simulink model "es2_emg_2"  (R2024a)
settings: Solver=VariableStepAuto  StartTime=0.0  StopTime=30  RelTol=1e-3
libraries: vrlib x2
settings Model: Creator=amisq  LastModifiedBy=amisq

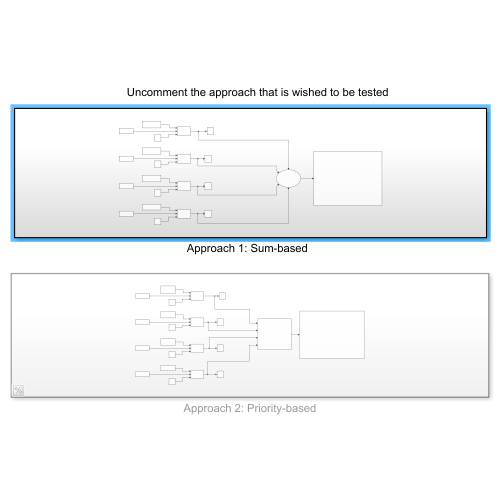
[thumbnail: Simulink's stored preview of the top-level diagram]
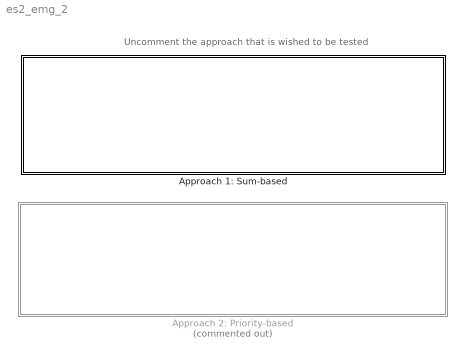
== system es2_emg_2 ==
  note: Uncomment the approach that is wished to be tested
  "Approach 1: Sum-based  " : Subsystem
  Approach 2: Priority-based : Subsystem  Commented=on

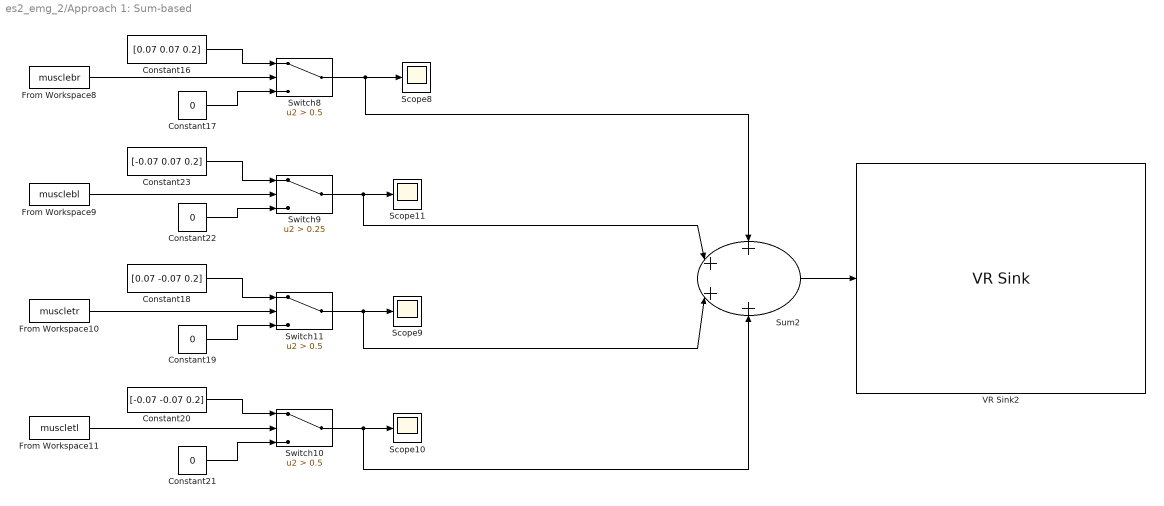
== system es2_emg_2/Approach 1: Sum-based   ==
  Constant16 : Constant  Value=[0.07 0.07 0.2]
  Constant{17,19,21..22} (4 alike) : Constant  Value=0
  Constant18 : Constant  Value=[0.07 -0.07 0.2]
  Constant20 : Constant  Value=[-0.07 -0.07 0.2]
  Constant23 : Constant  Value=[-0.07 0.07 0.2]
  From Workspace10 : FromWorkspace  VariableName=muscletr  SampleTime=0.05
  From Workspace11 : FromWorkspace  VariableName=muscletl  SampleTime=0.05
  From Workspace8 : FromWorkspace  VariableName=musclebr  SampleTime=0.05
  From Workspace9 : FromWorkspace  VariableName=musclebl  SampleTime=0.05
  Scope{8..11} (4 alike) : Scope
  Sum2 : Sum  Inputs=++++
  Switch10 : Switch  Criteria=u2 > Threshold  Threshold=0.5  SaturateOnIntegerOverflow=off  InputSameDT=off
  Switch11 : Switch  Criteria=u2 > Threshold  Threshold=0.5  SaturateOnIntegerOverflow=off  InputSameDT=off
  Switch8 : Switch  Criteria=u2 > Threshold  Threshold=0.5  SaturateOnIntegerOverflow=off  InputSameDT=off
  Switch9 : Switch  Criteria=u2 > Threshold  Threshold=0.25  SaturateOnIntegerOverflow=off  InputSameDT=off
  VR Sink2 : vrlib/VR Sink  InstantiateOnLoad=on  SampleTime=0.03  ViewEnable=on  RemoteChange=off  RemoteView=off  FieldsWritten=cursor.translation.3.1.1.double  WorldFileName=8_palline_color.wrl  AutoView=off  VideoDimensions=[]  AllowVariableSize=off
  wires:
  Constant19/1 -> Switch11/3
  Constant20/1 -> Switch10/1
  Constant21/1 -> Switch10/3
  From Workspace10/1 -> Switch11/2
  From Workspace8/1 -> Switch8/2
  Switch8/1 -> Sum2/1, Scope8/1
  From Workspace11/1 -> Switch10/2
  Switch10/1 -> Sum2/4, Scope10/1
  From Workspace9/1 -> Switch9/2
  Constant22/1 -> Switch9/3
  Sum2/1 -> VR Sink2/1
  Constant16/1 -> Switch8/1
  Switch9/1 -> Sum2/2, Scope11/1
  Constant18/1 -> Switch11/1
  Constant23/1 -> Switch9/1
  Switch11/1 -> Sum2/3, Scope9/1
  Constant17/1 -> Switch8/3

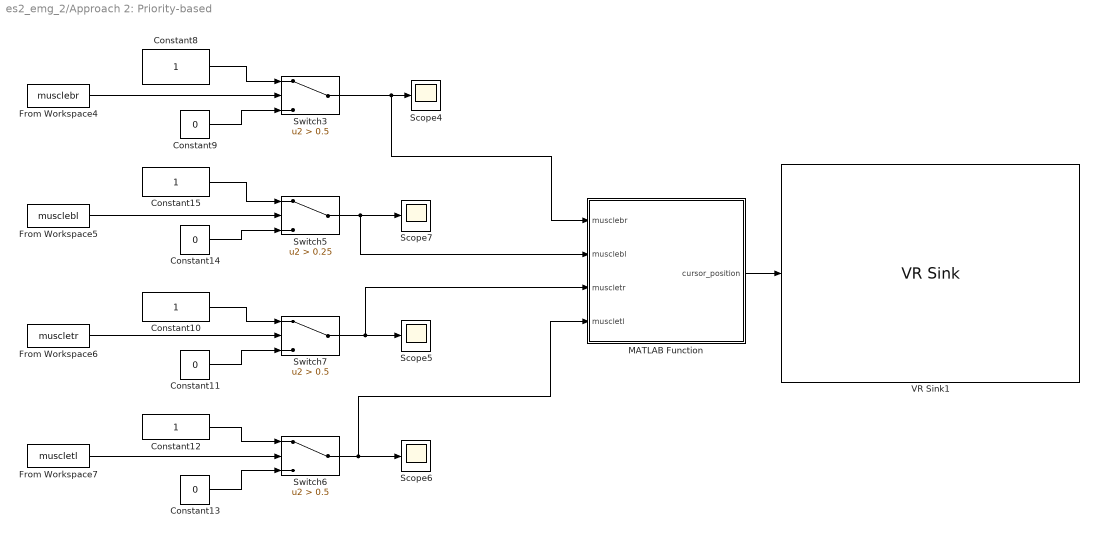
== system es2_emg_2/Approach 2: Priority-based ==
  Constant{8,10,12,15} (4 alike) : Constant
  Constant{9,11,13..14} (4 alike) : Constant  Value=0
  From Workspace4 : FromWorkspace  VariableName=musclebr  SampleTime=0.05
  From Workspace5 : FromWorkspace  VariableName=musclebl  SampleTime=0.05
  From Workspace6 : FromWorkspace  VariableName=muscletr  SampleTime=0.05
  From Workspace7 : FromWorkspace  VariableName=muscletl  SampleTime=0.05
  MATLAB Function : MATLAB Function  TreatAsAtomicUnit=on
  Scope{4..7} (4 alike) : Scope
  Switch3 : Switch  Criteria=u2 > Threshold  Threshold=0.5  SaturateOnIntegerOverflow=off  InputSameDT=off
  Switch5 : Switch  Criteria=u2 > Threshold  Threshold=0.25  SaturateOnIntegerOverflow=off  InputSameDT=off
  Switch6 : Switch  Criteria=u2 > Threshold  Threshold=0.5  SaturateOnIntegerOverflow=off  InputSameDT=off
  Switch7 : Switch  Criteria=u2 > Threshold  Threshold=0.5  SaturateOnIntegerOverflow=off  InputSameDT=off
  VR Sink1 : vrlib/VR Sink  InstantiateOnLoad=on  SampleTime=0.01  ViewEnable=on  RemoteChange=off  RemoteView=off  FieldsWritten=cursor.translation.3.1.1.double  WorldFileName=8_palline_color.wrl  AutoView=off  VideoDimensions=[]  AllowVariableSize=off
  wires:
  From Workspace4/1 -> Switch3/2
  From Workspace7/1 -> Switch6/2
  Switch6/1 -> MATLAB Function/4(muscletl), Scope6/1
  Constant11/1 -> Switch7/3
  MATLAB Function/1(cursor_position) -> VR Sink1/1
  Constant14/1 -> Switch5/3
  Constant15/1 -> Switch5/1
  Switch5/1 -> MATLAB Function/2(musclebl), Scope7/1
  Switch3/1 -> MATLAB Function/1(musclebr), Scope4/1
  Constant9/1 -> Switch3/3
  Constant12/1 -> Switch6/1
  Constant8/1 -> Switch3/1
  From Workspace5/1 -> Switch5/2
  Constant13/1 -> Switch6/3
  Switch7/1 -> Scope5/1, MATLAB Function/3(muscletr)
  From Workspace6/1 -> Switch7/2
  Constant10/1 -> Switch7/1

== matlab function es2_emg_2/Approach 2: Priority-based/MATLAB Function ==
  data: musclebr input; cursor_position output; musclebl input; muscletr input; muscletl input
function cursor_position = control_cursor(musclebr, musclebl, muscletr, muscletl)
    % Define the position vectors for the cardinal directions
    upright = [0.07, 0.07, 0.2];     % Muscle 1 (up)
    upleft = [-0.07, 0.07, 0.2];     % Muscle 2 (down)
    downright = [0.07, -0.07, 0.2];  % Muscle 3 (right)
    downleft = [-0.07, -0.07, 0.2];  % Muscle 4 (left)

    % Priority system: prioritize muscles in a specific order
    if musclebl
        cursor_position = upleft; % Priority 1: Up right
    elseif musclebr
        cursor_position = upright; % Priority 2: Up left 
    elseif muscletr
        cursor_position = downright; % Priority 3: Down right
    elseif muscletl
        cursor_position = downleft; % Priority 4: Down left
    else
        cursor_position = [0, 0, 0.2]; % No muscles active, no movement
    end
end
